simulink model "trainn_traction_system_4motors_CRH3_ver1"  (R2020b)
settings: Solver=VariableStepAuto  StartTime=0.0  StopTime=3  RelTol=1e-3
model workspace (MAT data in the model file):
  C = 0.016
  J = 5
  L = 0.005
  Llr = 0.006
  Lls = 0.001416
  Lm = 0.0254
  R = 0.2
  Rr = 0.16
  Rs = 0.15
  T = 1e-06
  Tloadmax = 100
  Tloadstart = 2
  Tpwm = 0.0001
  Ts = 0.0008
  Vdc_ref = 2700
  Vpeak = 1550
  f = 50
  noiseDense = 0.01
  np = 2
  sample_time = 2e-05
  tE1 = 3.25
  tE1w = 10
  tE2 = 10
  tE2w = 10
  tE3 = 10
  tE3w = 10
  tE4 = 10
  tE4w = 10
  t_precharge = 0.15
  w = 314.159265359
libraries: powerlib x19, simulink x19, pid_lib x1, eeSinusoidalMeasurementV2 x1
(part 1 of 3)
settings Model: SimulationMode=accelerator  OrderedModelArguments=off  Creator=messer  LastModifiedBy=messer

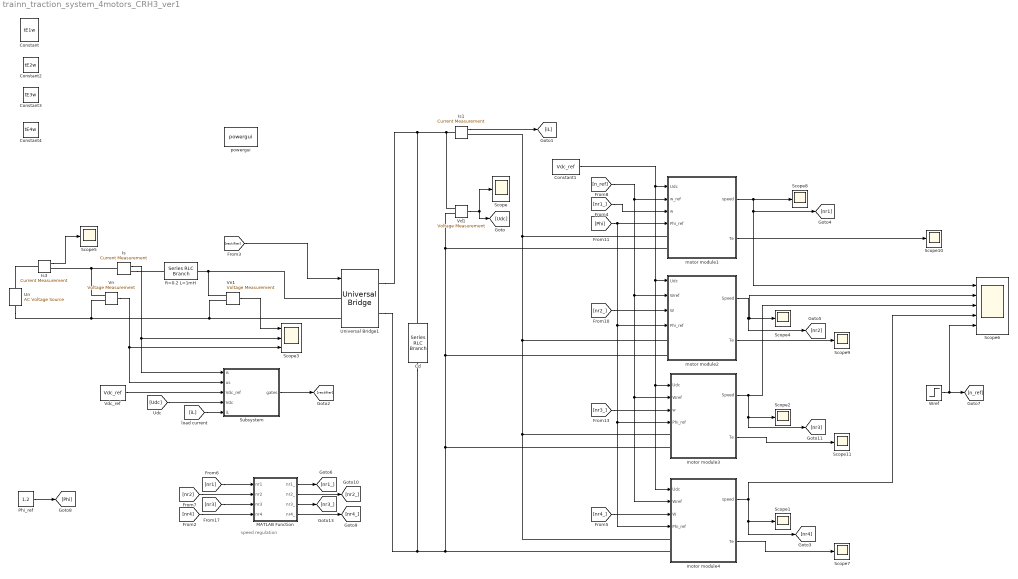
== system trainn_traction_system_4motors_CRH3_ver1 ==
  note: speed regulation
  Cd : powerlib/Elements/Series RLC Branch  LConnTagsString=__new0  RConnTagsString=__new0  BranchType=C  Resistance=1  Inductance=1e-3  SetiL0=off  InitialCurrent=0  Capacitance=C  Setx0=off  InitialVoltage=0  Measurements=None
  Constant : Constant  Value=tE1w
  Constant1 : Constant  Value=Vdc_ref
  Constant2 : Constant  Value=tE2w
  Constant3 : Constant  Value=tE3w
  Constant4 : Constant  Value=tE4w
  Is : powerlib/Measurements/Current Measurement  PhasorSimulation=off  OutputType=Complex  PSBequivalent=0
  Is1 : powerlib/Measurements/Current Measurement  PhasorSimulation=off  OutputType=Complex  PSBequivalent=0
  Is3 : powerlib/Measurements/Current Measurement  PhasorSimulation=off  OutputType=Complex  PSBequivalent=0
  MATLAB Function : MATLAB Function  TreatAsAtomicUnit=on
  Phi_ref : Constant  Value=1.2
  R=0.2 L=1mH : powerlib/Elements/Series RLC Branch  LConnTagsString=__new0  RConnTagsString=__new0  BranchType=RL  Resistance=R  Inductance=L  SetiL0=off  InitialCurrent=0  Capacitance=1e-6  Setx0=off  InitialVoltage=0  Measurements=None
  Scope{,1..2,4..5,7..11} (10 alike) : Scope
  Scope3 : Scope  NumInputPorts=3
  Scope6 : Scope  NumInputPorts=5
  Subsystem : Subsystem
  Un : powerlib/Electrical Sources/AC Voltage Source  Amplitude=Vpeak  Phase=0  Frequency=f  SampleTime=0  Measurements=None  BusType=swing  Pref=10e3  Qref=0  Qmin=-inf  Qmax=+inf
  Universal Bridge1 : powerlib/Power Electronics/Universal Bridge  Arms=2  SnubberResistance=1e5  SnubberCapacitance=inf  Device=IGBT / Diodes  Ron=1e-3  Lon=0  ForwardVoltages="[  0  0  ]"  ForwardVoltage=0  GTOparameters=[ 10e-6 , 20e-6 ]  IGBTparameters=[ 1e-6 , 2e-6 ]  Measurements=None  Measurements_2=None  converterType=Rectifier
  Vd1 : powerlib/Measurements/Voltage Measurement  PhasorSimulation=off  OutputType=Complex  PSBequivalent=0
  Vdc_ref : Constant  Value=Vdc_ref
  Vn : powerlib/Measurements/Voltage Measurement  PhasorSimulation=off  OutputType=Complex  PSBequivalent=0
  Vn1 : powerlib/Measurements/Voltage Measurement  PhasorSimulation=off  OutputType=Complex  PSBequivalent=0
  Wref : Step  Time=10  Before=1500  After=2000  SampleTime=0
  motor module1 : Subsystem
  motor module2 : Subsystem
  motor module3 : Subsystem
  motor module4 : Subsystem
  powergui : powerlib/powergui  Priority=1  SimulationMode=Discrete  SampleTime=T  frequency=60  Iterations=50  frequencyindice=0  Pbase=100e6  ErrMax=1e-4  UnitsV=kV  UnitsW=MW  buscounter=0  FunctionMessages=off  echomessages=off  EnableUseOfTLC=off  CurrentSourceSwitches=off  DisableSnubberDevices=off  DisableRonSwitches=off  DisableVfSwitches=off  DisplayEquations=off  AutomaticDiscreteSolvers=off  SolverType=Tustin/Backward Euler (TBE)  Interpol=off  ExternalGateDelay=off  methode=off  Ts=10  x0status=blocks  SPID=off  SwTol=0  HookPort=off  NonlinearTolerance=1e-4  nMaxIteration=100  ContinueOnMaxIteration=off  RestoreLinks=warning  ResistiveCurrentMeasurement=off  Frange=[0:2:500]  Ylog=off  Xlog=on  ShowGrid=off  save=off  variable=ZData  structure=0  ZoomFFT=off  StartTime=0.0  cycles=1  DisplayStyle=1  fundamental=60  FreqAxis=off  MaxFrequency=1000  frequencyindicesteady=1  RmsSteady=1  display=off
  wires:
  Is1/1 -> [iL]
  Vn/1 -> Subsystem/2(us), Scope3/3
  Is/1 -> Subsystem/1(is), Scope3/2
  Vn1/1 -> Scope3/1
  Vd1/1 -> Scope/1, [Udc]
  Vdc_ref/1 -> Subsystem/3(Vdc_ref)
  [Udc] -> Subsystem/4(Vdc)
  [iL] -> Subsystem/5(iL)
  [rectifier] -> Universal Bridge1/1
  Subsystem/1(gates) -> [rectifier]
  [nr1] -> MATLAB Function/1(nr1)
  Wref/1 -> Scope6/5, [n_ref]
  Phi_ref/1 -> [Phi]
  Is3/1 -> Scope5/1
  MATLAB Function/1(nr1_) -> [nr1_]
  MATLAB Function/2(nr2_) -> [nr2_]
  MATLAB Function/3(nr3_) -> [nr3_]
  Constant1/1 -> motor module4/1(Udc), motor module3/1(Udc), motor module2/1(Udc), motor module1/1(Udc)
  [n_ref] -> motor module4/2(Wref), motor module3/2(Wref), motor module2/2(Wref), motor module1/2(w_ref)
  [nr3_] -> motor module3/3(w)
  [Phi] -> motor module1/4(Phi_ref), motor module2/4(Phi_ref), motor module3/4(Phi_ref), motor module4/4(Phi_ref)
  motor module3/1(Speed) -> [nr3], Scope2/1, Scope6/3
  [nr2_] -> motor module2/3(W)
  motor module2/1(Speed) -> [nr2], Scope6/2, Scope4/1
  [nr1_] -> motor module1/3(w)
  motor module1/1(speed) -> Scope6/1, [nr1], Scope8/1
  motor module4/1(speed) -> Scope1/1, [nr4], Scope6/4
  MATLAB Function/4(nr4_) -> [nr4_]
  [nr4_] -> motor module4/3(W)
  [nr2] -> MATLAB Function/2(nr2)
  [nr3] -> MATLAB Function/3(nr3)
  [nr4] -> MATLAB Function/4(nr4)
  motor module1/2(Te) -> Scope10/1
  motor module2/2(Te) -> Scope9/1
  motor module3/2(Te) -> Scope11/1
  motor module4/2(Te) -> Scope7/1
  connections:
  motor module3/LConn1 -- motor module4/LConn1 -- motor module2/LConn1 -- motor module1/LConn1 -- Is1/RConn1
  Is3/RConn1 -- Is/LConn1 -- Vn/LConn1
  Cd/RConn1 -- Vd1/LConn2 -- motor module1/LConn2 -- motor module2/LConn2 -- motor module3/LConn2 -- motor module4/LConn2 -- Universal Bridge1/RConn2
  Universal Bridge1/LConn1 -- R=0.2 L=1mH/RConn1 -- Vn1/LConn1
  Vn1/LConn2 -- Un/LConn1 -- Vn/LConn2 -- Universal Bridge1/LConn2
  Vd1/LConn1 -- Universal Bridge1/RConn1 -- Cd/LConn1 -- Is1/LConn1
  Is/RConn1 -- R=0.2 L=1mH/LConn1
  Is3/LConn1 -- Un/RConn1

== system trainn_traction_system_4motors_CRH3_ver1/Subsystem ==
  is : Inport
  us : Inport  Port=2
  Vdc_ref : Inport  Port=3
  Vdc : Inport  Port=4
  iL : Inport  Port=5
  Gain : Gain  Gain=2/Vpeak
  Gain1 : Gain  Gain=R
  Gain2 : Gain  Gain=w*L
  Gain4 : Gain
  PID Controller : pid_lib/PID Controller  Controller=PI  Form=Parallel  TimeDomain=Continuous-time  UseExternalTs=off  SampleTime=-1  IntegratorMethod=Forward Euler  FilterMethod=Forward Euler  ControllerParametersSource=internal  P=11  I=0.13  D=0  UseFilter=on  N=100  TunerSelectOption=Transfer Function Based (PID Tuner App)  InitialConditionSource=internal  InitialConditionForIntegrator=0  InitialConditionForFilter=0  DifferentiatorICPrevScaledInput=0  ExternalReset=none  TrackingMode=off  Kt=1  LimitOutput=off  SatLimitsSource=internal  UpperSaturationLimit=inf  LowerSaturationLimit=-inf  LinearizeAsGain=on  AntiWindupMode=none  Kb=1  POutMin=[]  POutMax=[]  IOutMin=[]  IOutMax=[]  DOutMin=[]  DOutMax=[]  NOutMin=[]  NOutMax=[]  SumOutMin=[]  SumOutMax=[]  SaturationOutMin=[]  SaturationOutMax=[]  PParamMin=[]  PParamMax=[]  IParamMin=[]  IParamMax=[]  DParamMin=[]  DParamMax=[]  NParamMin=[]  NParamMax=[]  KbParamMin=[]  KbParamMax=[]  KtParamMin=[]  KtParamMax=[]  KbOutMin=[]  KbOutMax=[]  KtOutMin=[]  KtOutMax=[]  IntegratorOutMin=[]  IntegratorOutMax=[]  FilterOutMin=[]  FilterOutMax=[]  SumI1OutMin=[]  SumI1OutMax=[]  SumI2OutMin=[]  SumI2OutMax=[]  SumI3OutMin=[]  SumI3OutMax=[]  SumI4OutMin=[]  SumI4OutMax=[]  SumDOutMin=[]  SumDOutMax=[]  DifferentiatorOutMin=[]  DifferentiatorOutMax=[]  FilterDiffOutCoefMin=[]  FilterDiffOutCoefMax=[]  ReciprocalOutMin=[]  ReciprocalOutMax=[]  SumDenOutMin=[]  SumDenOutMax=[]  SumNumOutMin=[]  SumNumOutMax=[]  DivideOutMin=[]  DivideOutMax=[]  UdiffTsProdOutMin=[]  UdiffTsProdOutMax=[]  NTsProdOutMin=[]  NTsProdOutMax=[]  UintegralTsProdOutMin=[]  UintegralTsProdOutMax=[]  UngainTsProdOutMin=[]  UngainTsProdOutMax=[]  IntegratorContinuousStateAttributes=''  IntegratorStateMustResolveToSignalObject=off  IntegratorRTWStateStorageClass=Auto  FilterContinuousStateAttributes=''  FilterStateMustResolveToSignalObject=off  FilterRTWStateStorageClass=Auto  ParallelPVariant=InternalParameters  IdealPVariant=Disabled  IVariant=InternalParameters  DVariant=Disabled  IntegratorVariant=Continuous  SatVariant=Disabled  AWVariant=Passthrough  PCopyVariant=Disabled  TRVariant=Disabled  FdbkBlocksVariant=Forward  IdealPFdbkVariant=Disabled  SatFdbkVariant=Disabled  DerivativeFilterVariant=Disabled  NVariant=Disabled  NCopyVariant=Disabled_SignalSpec  FilterICVariant=Disabled  IntegratorICVariant=InternalICs  ExternalResetVariant=Disabled  TRSumVariant=Passthrough  SumFdbkVariant=Disabled  SumVariant=Sum_PI  TsampFilterVariant=InternalTs  TsampNgainVariant=Passthrough  TsampIntegralVariant=Passthrough  ExternalSaturationOutDataTypeStr=Inherit: Same as second input
  Product : Product
  Product1 : Product
  Product2 : Product
  SinCos : Trigonometry  Operator=sincos
  Sinusoidal Measurement (PLL) : eeSinusoidalMeasurementV2/Sinusoidal Measurement (PLL)  Ki_PD=1000  Kp_LF=400  Ki_LF=20000  F0=60  Theta0=0  Mag0=1  Ts=-1
      settings: SourceProductBaseCode=PS
  Sum : Sum  Inputs=|+-
  Sum1 : Sum  Inputs=|++
  Sum2 : Sum  Inputs=+-|--
  Sum9 : Sum  Inputs=-+|
  gen_trigger : Subsystem
  gates : Outport
  wires:
  Sum1/1 -> Product2/2, Product1/2
  SinCos/2 -> Product2/1
  SinCos/1 -> Product1/1
  Gain/1 -> Sum1/2
  Sum/1 -> PID Controller/1
  Vdc/1 -> Product/1, Sum/2
  Product1/1 -> Sum9/2, Gain1/1
  PID Controller/1 -> Sum1/1
  Product/1 -> Gain/1
  Product2/1 -> Gain2/1
  Sinusoidal Measurement (PLL)/2 -> SinCos/1
  Gain2/1 -> Sum2/4
  is/1 -> Sum2/1, Sum9/1
  iL/1 -> Product/2
  Sum2/1 -> gen_trigger/1(uab)
  Gain4/1 -> Sum2/2
  Gain1/1 -> Sum2/3
  Sum9/1 -> Gain4/1
  us/1 -> Sinusoidal Measurement (PLL)/1
  gen_trigger/1(gates) -> gates/1
  Vdc_ref/1 -> Sum/1

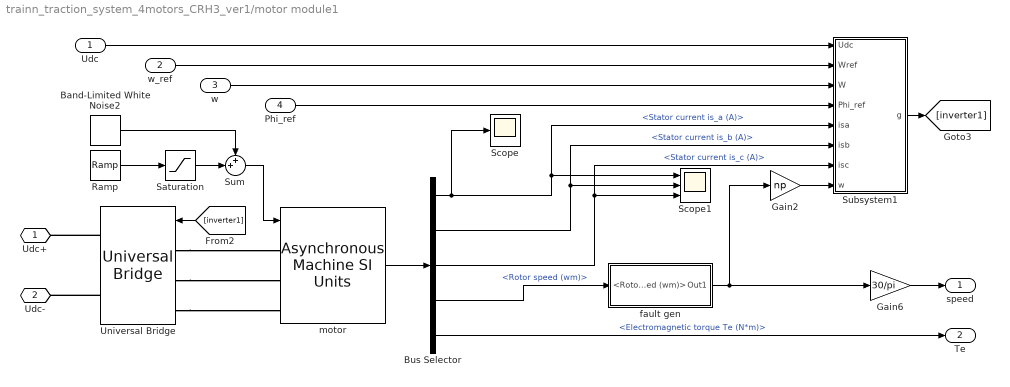
== system trainn_traction_system_4motors_CRH3_ver1/motor module1 ==
  Udc : Inport
  w_ref : Inport  Port=2
  w : Inport  Port=3
  Phi_ref : Inport  Port=4
  Band-Limited White Noise2 : simulink/Sources/Band-Limited White Noise  Cov=[0.0001]  Ts=1e-4  seed=[130341]
  Bus Selector : BusSelector  OutputSignals=Stator measurements.Stator current is_a (A),Stator measurements.Stator current is_b (A),Stator measurements.Stator current is_c (A),Mechanical.Rotor speed (wm),Mechanical.Electromagnetic torque Te (N*m)
  Gain2 : Gain  Gain=np
  Gain6 : Gain  Gain=30/pi
  Ramp : simulink/Sources/Ramp  slope=240  start=Tloadstart  InitialOutput=0
  Saturation : Saturate  UpperLimit=Tloadmax  LowerLimit=0
  Scope : Scope
  Scope1 : Scope  NumInputPorts=3
  Subsystem1 : Subsystem
  Sum : Sum  Inputs=++|
  Universal Bridge : powerlib/Power Electronics/Universal Bridge  Arms=3  SnubberResistance=1e5  SnubberCapacitance=inf  Device=IGBT / Diodes  Ron=1e-3  Lon=0  ForwardVoltages="[  0  0  ]"  ForwardVoltage=0  GTOparameters=[ 10e-6 , 20e-6 ]  IGBTparameters=[ 1e-6 , 2e-6 ]  Measurements=None  Measurements_2=None  converterType=Rectifier
  fault gen : Subsystem
  motor : powerlib/Machines/Asynchronous Machine SI Units  RotorType=Squirrel-cage  PresetModel=No  MechanicalLoad=Torque Tm  ShowDetailedParameters=on  ReferenceFrame=Stationary  Units=SI  MeasurementBus=off  NominalParameters=[562000 2750 135]  Stator=[1.02136*Rs 0.808987*Lls]  Rotor=[0.95069*Rr 0.92145*Llr]  Cage1=[0.4155 0.002066]  Cage2=[0.4168 0.0003495]  Lm=0.88963*Lm  Mechanical=[0.97052*J 0 np]  PolePairs=2  InitialConditions=[1 0 0 0 0 0 0 0]  SimulateSaturation=off  Saturation=[14.03593122, 27.81365428, 53.79336849, 72.68890987, 97.98006896, 148.6815601, 215.7428561, 302.9841135, 428.7778367 ; 230, 322, 414, 460, 506, 552, 598, 644, 690]  LoadFlowParameters=1492000  TsPowergui=0  TsBlock=-1  IterativeModel=Trapezoidal non iterative  IterativeDiscreteModel=Trapezoidal non iterative  Pmec=1.492e+006
  Udc+ : PMIOPort  Side=Left
  Udc- : PMIOPort  Port=2  Side=Left
  speed : Outport
  Te : Outport  Port=2
  wires:
  Gain6/1 -> speed/1
  Subsystem1/1(g) -> [inverter1]
  Bus Selector/1 -> Scope/1, Subsystem1/5(isa), Scope1/1  "<Stator current is_a (A)>"
  Bus Selector/2 -> Subsystem1/6(isb), Scope1/2  "<Stator current is_b (A)>"
  motor/1 -> Bus Selector/1
  Gain2/1 -> Subsystem1/8(w)
  Bus Selector/3 -> Subsystem1/7(isc), Scope1/3  "<Stator current is_c (A)>"
  Bus Selector/5 -> Te/1  "<Electromagnetic torque Te (N*m)>"
  [inverter1] -> Universal Bridge/1
  Udc/1 -> Subsystem1/1(Udc)
  w/1 -> Subsystem1/3(W)
  Phi_ref/1 -> Subsystem1/4(Phi_ref)
  w_ref/1 -> Subsystem1/2(Wref)
  Ramp/1 -> Saturation/1
  Saturation/1 -> Sum/2
  Band-Limited White Noise2/1 -> Sum/1
  Sum/1 -> motor/1
  fault gen/1(Out1) -> Gain6/1, Gain2/1
  Bus Selector/4 -> fault gen/1(<Rotor speed (wm)>)  "<Rotor speed (wm)>"
  connections:
  Universal Bridge/LConn2 -- motor/LConn2
  Universal Bridge/LConn1 -- motor/LConn1
  Universal Bridge/LConn3 -- motor/LConn3
  Universal Bridge/RConn2 -- Udc-/RConn1
  Universal Bridge/RConn1 -- Udc+/RConn1

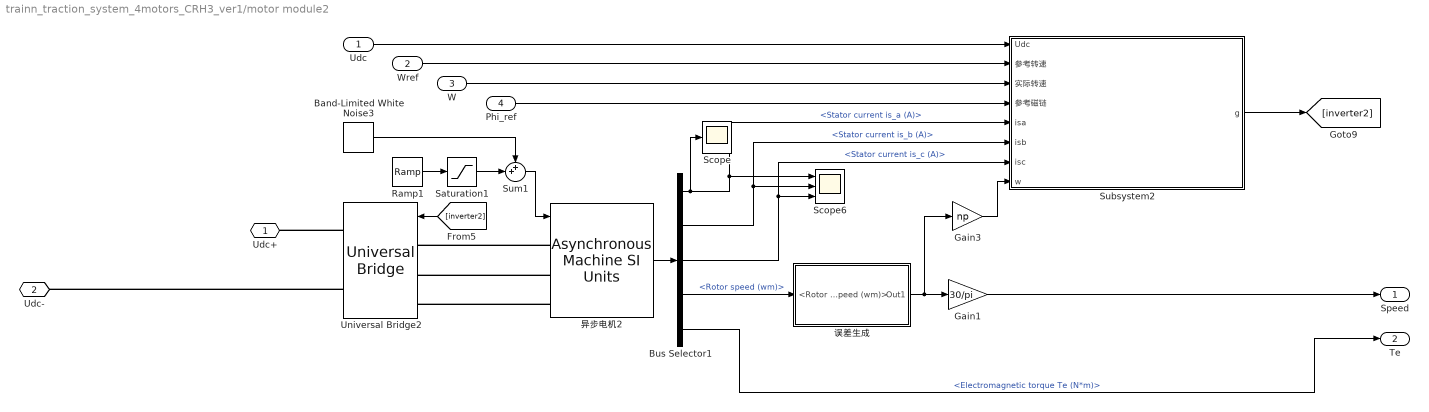
== system trainn_traction_system_4motors_CRH3_ver1/motor module2 ==
  Udc : Inport
  Wref : Inport  Port=2
  W : Inport  Port=3
  Phi_ref : Inport  Port=4
  Band-Limited White Noise3 : simulink/Sources/Band-Limited White Noise  Cov=[0.0001]  Ts=1e-4  seed=[130341]
  Bus Selector1 : BusSelector  OutputSignals=Stator measurements.Stator current is_a (A),Stator measurements.Stator current is_b (A),Stator measurements.Stator current is_c (A),Mechanical.Rotor speed (wm),Mechanical.Electromagnetic torque Te (N*m)
  Gain1 : Gain  Gain=30/pi
  Gain3 : Gain  Gain=np
  Ramp1 : simulink/Sources/Ramp  slope=240  start=Tloadstart  InitialOutput=0
  Saturation1 : Saturate  UpperLimit=Tloadmax  LowerLimit=0
  Scope : Scope
  Scope6 : Scope  NumInputPorts=3
  Subsystem2 : Subsystem
  Sum1 : Sum  Inputs=++|
  Universal Bridge2 : powerlib/Power Electronics/Universal Bridge  Arms=3  SnubberResistance=1e5  SnubberCapacitance=inf  Device=IGBT / Diodes  Ron=1e-3  Lon=0  ForwardVoltages="[  0  0  ]"  ForwardVoltage=0  GTOparameters=[ 10e-6 , 20e-6 ]  IGBTparameters=[ 1e-6 , 2e-6 ]  Measurements=None  Measurements_2=None  converterType=Rectifier
  异步电机2 : powerlib/Machines/Asynchronous Machine SI Units  RotorType=Squirrel-cage  PresetModel=No  MechanicalLoad=Torque Tm  ShowDetailedParameters=on  ReferenceFrame=Stationary  Units=SI  MeasurementBus=off  NominalParameters=[562000 2750 135]  Stator=[1.09135*Rs 0.864431*Lls]  Rotor=[0.9864*Rr 0.92145*Llr]  Cage1=[0.4155 0.002066]  Cage2=[0.4168 0.0003495]  Lm=Lm*1.03442  Mechanical=[1.054266*J 0 np]  PolePairs=2  InitialConditions=[1 0 0 0 0 0 0 0]  SimulateSaturation=off  Saturation=[14.03593122, 27.81365428, 53.79336849, 72.68890987, 97.98006896, 148.6815601, 215.7428561, 302.9841135, 428.7778367 ; 230, 322, 414, 460, 506, 552, 598, 644, 690]  LoadFlowParameters=1492000  TsPowergui=0  TsBlock=-1  IterativeModel=Trapezoidal non iterative  IterativeDiscreteModel=Trapezoidal non iterative  Pmec=1.492e+006
  误差生成 : Subsystem
  Udc+ : PMIOPort  Side=Left
  Udc- : PMIOPort  Port=2  Side=Left
  Speed : Outport
  Te : Outport  Port=2
  wires:
  Bus Selector1/2 -> Subsystem2/6(isb), Scope6/2  "<Stator current is_b (A)>"
  异步电机2/1 -> Bus Selector1/1
  Bus Selector1/4 -> 误差生成/1(<Rotor speed (wm)>)  "<Rotor speed (wm)>"
  W/1 -> Subsystem2/3(实际转速)
  Gain1/1 -> Speed/1
  Bus Selector1/3 -> Subsystem2/7(isc), Scope6/3  "<Stator current is_c (A)>"
  [inverter2] -> Universal Bridge2/1
  Subsystem2/1(g) -> [inverter2]
  Gain3/1 -> Subsystem2/8(w)
  Udc/1 -> Subsystem2/1(Udc)
  Bus Selector1/1 -> Scope/1, Subsystem2/5(isa), Scope6/1  "<Stator current is_a (A)>"
  Bus Selector1/5 -> Te/1  "<Electromagnetic torque Te (N*m)>"
  Phi_ref/1 -> Subsystem2/4(参考磁链)
  Wref/1 -> Subsystem2/2(参考转速)
  误差生成/1(Out1) -> Gain3/1, Gain1/1
  Band-Limited White Noise3/1 -> Sum1/1
  Ramp1/1 -> Saturation1/1
  Saturation1/1 -> Sum1/2
  Sum1/1 -> 异步电机2/1
  connections:
  异步电机2/LConn2 -- Universal Bridge2/LConn2
  异步电机2/LConn1 -- Universal Bridge2/LConn1
  异步电机2/LConn3 -- Universal Bridge2/LConn3
  Universal Bridge2/RConn2 -- Udc-/RConn1
  Universal Bridge2/RConn1 -- Udc+/RConn1

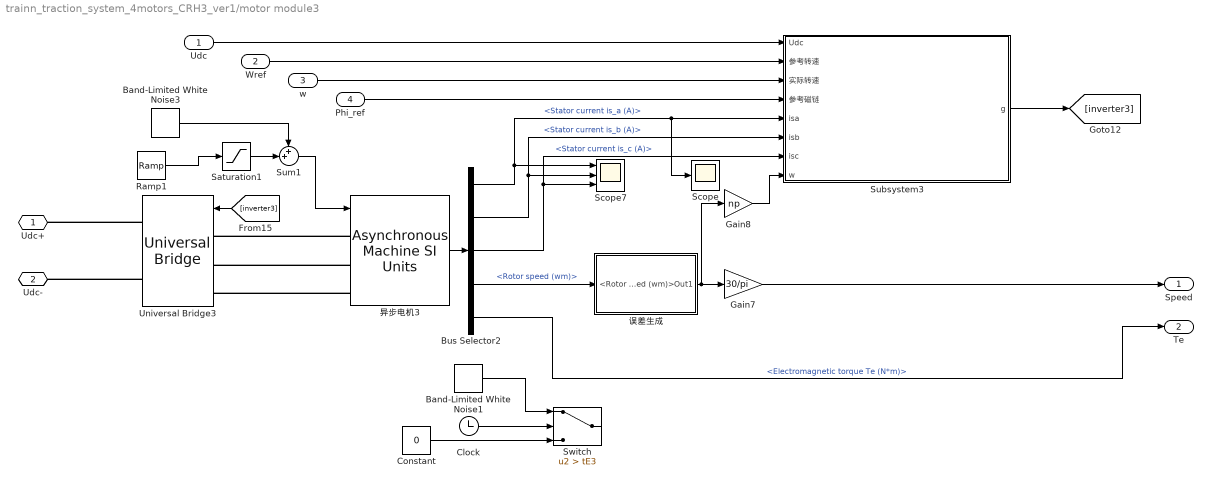
== system trainn_traction_system_4motors_CRH3_ver1/motor module3 ==
  Udc : Inport
  Wref : Inport  Port=2
  w : Inport  Port=3
  Phi_ref : Inport  Port=4
  Band-Limited White Noise1 : simulink/Sources/Band-Limited White Noise  Cov=[0.11]  Ts=noiseDense  seed=[23341]
  Band-Limited White Noise3 : simulink/Sources/Band-Limited White Noise  Cov=[0.0001]  Ts=1e-4  seed=[130341]
  Bus Selector2 : BusSelector  OutputSignals=Stator measurements.Stator current is_a (A),Stator measurements.Stator current is_b (A),Stator measurements.Stator current is_c (A),Mechanical.Rotor speed (wm),Mechanical.Electromagnetic torque Te (N*m)
  Clock : Clock
  Constant : Constant  Value=0
  Gain7 : Gain  Gain=30/pi
  Gain8 : Gain  Gain=np
  Ramp1 : simulink/Sources/Ramp  slope=240  start=Tloadstart  InitialOutput=0
  Saturation1 : Saturate  UpperLimit=Tloadmax  LowerLimit=0
  Scope : Scope
  Scope7 : Scope  NumInputPorts=3
  Subsystem3 : Subsystem
  Sum1 : Sum  Inputs=++|
  Switch : Switch  Criteria=u2 > Threshold  Threshold=tE3
  Universal Bridge3 : powerlib/Power Electronics/Universal Bridge  Arms=3  SnubberResistance=1e5  SnubberCapacitance=inf  Device=IGBT / Diodes  Ron=1e-3  Lon=0  ForwardVoltages="[  0  0  ]"  ForwardVoltage=0  GTOparameters=[ 10e-6 , 20e-6 ]  IGBTparameters=[ 1e-6 , 2e-6 ]  Measurements=None  Measurements_2=None  converterType=Rectifier
  异步电机3 : powerlib/Machines/Asynchronous Machine SI Units  RotorType=Squirrel-cage  PresetModel=No  MechanicalLoad=Torque Tm  ShowDetailedParameters=on  ReferenceFrame=Stationary  Units=SI  MeasurementBus=off  NominalParameters=[562000 2750 135]  Stator=[0.9819810*Rs Lls*0.832368]  Rotor=[0.978836*Rr Llr*1.00113]  Cage1=[0.4155 0.002066]  Cage2=[0.4168 0.0003495]  Lm=Lm*0.938915  Mechanical=[0.98615*J 0 np]  PolePairs=2  InitialConditions=[1 0 0 0 0 0 0 0]  SimulateSaturation=off  Saturation=[14.03593122, 27.81365428, 53.79336849, 72.68890987, 97.98006896, 148.6815601, 215.7428561, 302.9841135, 428.7778367 ; 230, 322, 414, 460, 506, 552, 598, 644, 690]  LoadFlowParameters=1492000  TsPowergui=0  TsBlock=-1  IterativeModel=Trapezoidal non iterative  IterativeDiscreteModel=Trapezoidal non iterative  Pmec=1.492e+006
  误差生成 : Subsystem
  Udc+ : PMIOPort  Side=Left
  Udc- : PMIOPort  Port=2  Side=Left
  Speed : Outport
  Te : Outport  Port=2
  wires:
  Bus Selector2/1 -> Scope/1, Subsystem3/5(isa), Scope7/1  "<Stator current is_a (A)>"
  Bus Selector2/4 -> 误差生成/1(<Rotor speed (wm)>)  "<Rotor speed (wm)>"
  Subsystem3/1(g) -> [inverter3]
  Gain7/1 -> Speed/1
  Bus Selector2/5 -> Te/1  "<Electromagnetic torque Te (N*m)>"
  Bus Selector2/3 -> Scope7/3, Subsystem3/7(isc)  "<Stator current is_c (A)>"
  Wref/1 -> Subsystem3/2(参考转速)
  Gain8/1 -> Subsystem3/8(w)
  [inverter3] -> Universal Bridge3/1
  Bus Selector2/2 -> Subsystem3/6(isb), Scope7/2  "<Stator current is_b (A)>"
  异步电机3/1 -> Bus Selector2/1
  w/1 -> Subsystem3/3(实际转速)
  Phi_ref/1 -> Subsystem3/4(参考磁链)
  Udc/1 -> Subsystem3/1(Udc)
  Band-Limited White Noise1/1 -> Switch/1
  Constant/1 -> Switch/3
  Clock/1 -> Switch/2
  误差生成/1(Out1) -> Gain8/1, Gain7/1
  Band-Limited White Noise3/1 -> Sum1/1
  Ramp1/1 -> Saturation1/1
  Saturation1/1 -> Sum1/2
  Sum1/1 -> 异步电机3/1
  connections:
  异步电机3/LConn1 -- Universal Bridge3/LConn1
  异步电机3/LConn3 -- Universal Bridge3/LConn3
  异步电机3/LConn2 -- Universal Bridge3/LConn2
  Universal Bridge3/RConn1 -- Udc+/RConn1
  Universal Bridge3/RConn2 -- Udc-/RConn1

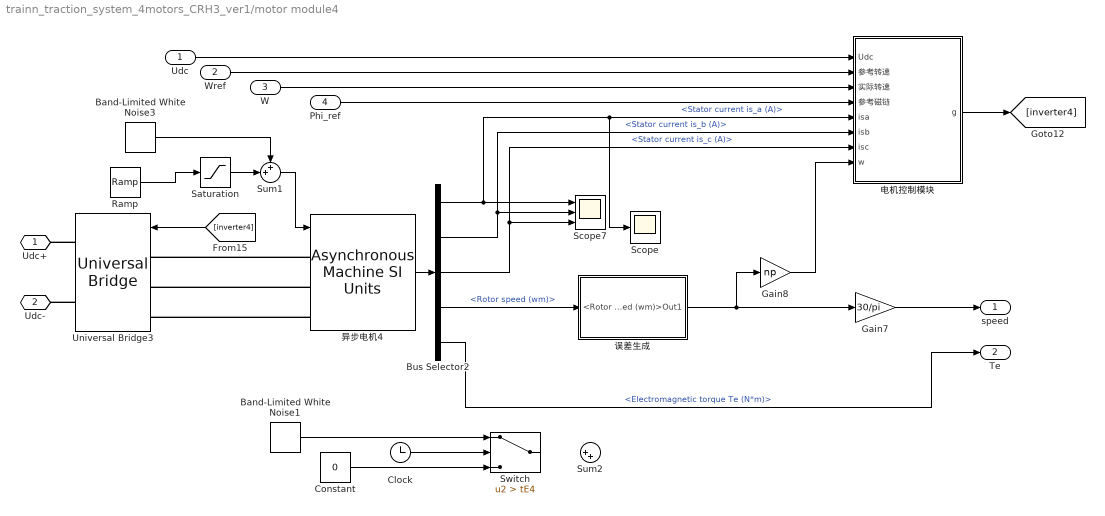
== system trainn_traction_system_4motors_CRH3_ver1/motor module4 ==
  Udc : Inport
  Wref : Inport  Port=2
  W : Inport  Port=3
  Phi_ref : Inport  Port=4
  Band-Limited White Noise1 : simulink/Sources/Band-Limited White Noise  Cov=[0.11]  Ts=noiseDense  seed=[23341]
  Band-Limited White Noise3 : simulink/Sources/Band-Limited White Noise  Cov=[0.0001]  Ts=1e-4  seed=[130341]
  Bus Selector2 : BusSelector  OutputSignals=Stator measurements.Stator current is_a (A),Stator measurements.Stator current is_b (A),Stator measurements.Stator current is_c (A),Mechanical.Rotor speed (wm),Mechanical.Electromagnetic torque Te (N*m)
  Clock : Clock
  Constant : Constant  Value=0
  Gain7 : Gain  Gain=30/pi
  Gain8 : Gain  Gain=np
  Ramp : simulink/Sources/Ramp  slope=240  start=Tloadstart  InitialOutput=0
  Saturation : Saturate  UpperLimit=Tloadmax  LowerLimit=0
  Scope : Scope
  Scope7 : Scope  NumInputPorts=3
  Sum1 : Sum  Inputs=++|
  Sum2 : Sum  Inputs=|++
  Switch : Switch  Criteria=u2 > Threshold  Threshold=tE4
  Universal Bridge3 : powerlib/Power Electronics/Universal Bridge  Arms=3  SnubberResistance=1e5  SnubberCapacitance=inf  Device=IGBT / Diodes  Ron=1e-3  Lon=0  ForwardVoltages="[  0  0  ]"  ForwardVoltage=0  GTOparameters=[ 10e-6 , 20e-6 ]  IGBTparameters=[ 1e-6 , 2e-6 ]  Measurements=None  Measurements_2=None  converterType=Rectifier
  异步电机4 : powerlib/Machines/Asynchronous Machine SI Units  RotorType=Squirrel-cage  PresetModel=No  MechanicalLoad=Torque Tm  ShowDetailedParameters=on  ReferenceFrame=Stationary  Units=SI  MeasurementBus=off  NominalParameters=[562000 2750 135]  Stator=[1.02136*Rs Lls*0.8933278]  Rotor=[1.01302*Rr Llr*1.037898]  Cage1=[0.4155 0.002066]  Cage2=[0.4168 0.0003495]  Lm=Lm*1.00281  Mechanical=[0.97849*J 0 np]  PolePairs=2  InitialConditions=[1 0 0 0 0 0 0 0]  SimulateSaturation=off  Saturation=[14.03593122, 27.81365428, 53.79336849, 72.68890987, 97.98006896, 148.6815601, 215.7428561, 302.9841135, 428.7778367 ; 230, 322, 414, 460, 506, 552, 598, 644, 690]  LoadFlowParameters=1492000  TsPowergui=0  TsBlock=-1  IterativeModel=Trapezoidal non iterative  IterativeDiscreteModel=Trapezoidal non iterative  Pmec=1.492e+006
  电机控制模块 : Subsystem
  误差生成 : Subsystem
  Udc+ : PMIOPort  Side=Left
  Udc- : PMIOPort  Port=2  Side=Left
  speed : Outport
  Te : Outport  Port=2
  wires:
  Udc/1 -> 电机控制模块/1(Udc)
  Phi_ref/1 -> 电机控制模块/4(参考磁链)
  W/1 -> 电机控制模块/3(实际转速)
  异步电机4/1 -> Bus Selector2/1
  Bus Selector2/2 -> 电机控制模块/6(isb), Scope7/2  "<Stator current is_b (A)>"
  [inverter4] -> Universal Bridge3/1
  Gain8/1 -> 电机控制模块/8(w)
  Wref/1 -> 电机控制模块/2(参考转速)
  Bus Selector2/3 -> 电机控制模块/7(isc), Scope7/3  "<Stator current is_c (A)>"
  Bus Selector2/5 -> Te/1  "<Electromagnetic torque Te (N*m)>"
  Gain7/1 -> speed/1
  电机控制模块/1(g) -> [inverter4]
  Bus Selector2/4 -> 误差生成/1(<Rotor speed (wm)>)  "<Rotor speed (wm)>"
  Bus Selector2/1 -> Scope/1, 电机控制模块/5(isa), Scope7/1  "<Stator current is_a (A)>"
  Constant/1 -> Switch/3
  Clock/1 -> Switch/2
  Band-Limited White Noise1/1 -> Switch/1
  误差生成/1(Out1) -> Gain7/1, Gain8/1
  Band-Limited White Noise3/1 -> Sum1/1
  Ramp/1 -> Saturation/1
  Saturation/1 -> Sum1/2
  Sum1/1 -> 异步电机4/1
  connections:
  Universal Bridge3/RConn2 -- Udc-/RConn1
  Universal Bridge3/RConn1 -- Udc+/RConn1
  异步电机4/LConn2 -- Universal Bridge3/LConn2
  异步电机4/LConn3 -- Universal Bridge3/LConn3
  异步电机4/LConn1 -- Universal Bridge3/LConn1

== system trainn_traction_system_4motors_CRH3_ver1/Subsystem/gen_trigger ==
  uab : Inport
  Gain4 : Gain  Gain=1/Vdc_ref
  Gain5 : Gain  Gain=-1
  Mux : Mux
  NOT : Logic  Operator=NOT  IconShape=distinctive  AllPortsSameDT=off  OutDataTypeStr=boolean
  NOT1 : Logic  Operator=NOT  IconShape=distinctive  AllPortsSameDT=off  OutDataTypeStr=boolean
  Relational Operator : RelationalOperator  OutDataTypeStr=boolean  RndMeth=Simplest
  Relational Operator1 : RelationalOperator  OutDataTypeStr=boolean  RndMeth=Simplest
  Repeating Sequence : simulink/Sources/Repeating Sequence  rep_seq_t=[0 Ts/2 Ts]  rep_seq_y=[-1 1 -1]
  gates : Outport
  wires:
  Relational Operator1/1 -> NOT1/1, Mux/3
  Repeating Sequence/1 -> Relational Operator1/2, Relational Operator/2
  Gain4/1 -> Relational Operator/1, Gain5/1
  NOT/1 -> Mux/2
  uab/1 -> Gain4/1
  Relational Operator/1 -> NOT/1, Mux/1
  Mux/1 -> gates/1
  Gain5/1 -> Relational Operator1/1
  NOT1/1 -> Mux/4

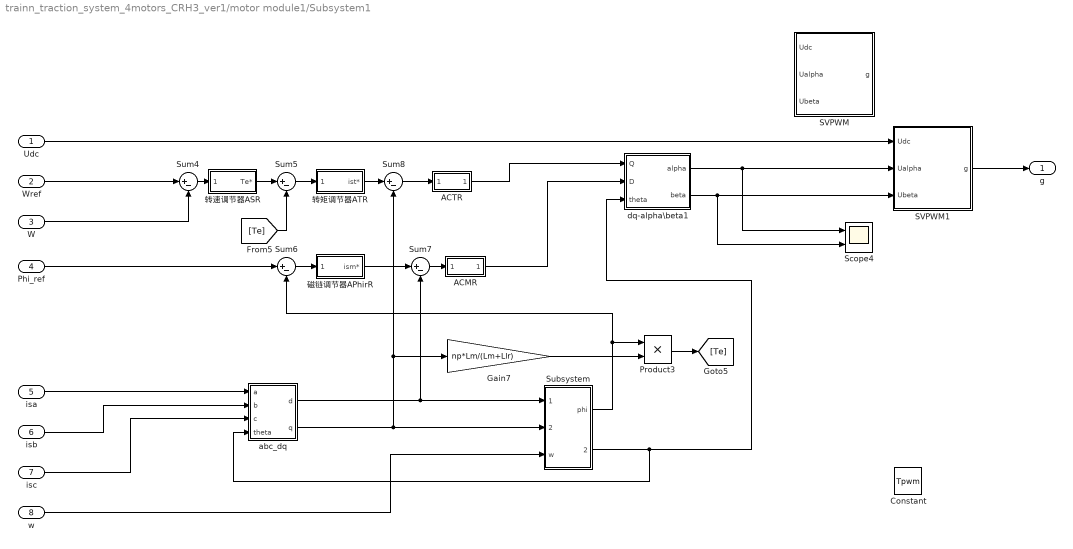
== system trainn_traction_system_4motors_CRH3_ver1/motor module1/Subsystem1 ==
  Udc : Inport
  Wref : Inport  Port=2
  W : Inport  Port=3
  Phi_ref : Inport  Port=4
  isa : Inport  Port=5
  isb : Inport  Port=6
  isc : Inport  Port=7
  w : Inport  Port=8
  ACMR : Subsystem
  ACTR : Subsystem
  Constant : Constant  Value=Tpwm
  Gain7 : Gain  Gain=np*Lm/(Lm+Llr)
  Product3 : Product
  SVPWM : Subsystem
  SVPWM1 : Subsystem
  Scope4 : Scope  NumInputPorts=2
  Subsystem : Subsystem
  Sum{4..8} (5 alike) : Sum  Inputs=|+-
  abc_dq : Subsystem
  dq-alpha\beta1 : Subsystem
  磁链调节器APhirR : Subsystem
  转矩调节器ATR : Subsystem
  转速调节器ASR : Subsystem
  g : Outport
  wires:
  磁链调节器APhirR/1(ism*) -> Sum7/1
  dq-alpha\beta1/1(alpha) -> SVPWM1/2(Ualpha), Scope4/1
  Wref/1 -> Sum4/1
  ACMR/1(" ") -> dq-alpha\beta1/2(D)
  isa/1 -> abc_dq/1(a)
  Sum8/1 -> ACTR/1("  ")
  Subsystem/1(phi) -> Sum6/2, Product3/1
  Subsystem/2(theta) -> abc_dq/4(theta), dq-alpha\beta1/3(theta)
  Gain7/1 -> Product3/2
  W/1 -> Sum4/2
  Product3/1 -> [Te]
  Sum7/1 -> ACMR/1("  ")
  Sum6/1 -> 磁链调节器APhirR/1(" ")
  转矩调节器ATR/1(ist*) -> Sum8/1
  [Te] -> Sum5/2
  转速调节器ASR/1(Te*) -> Sum5/1
  ACTR/1(" ") -> dq-alpha\beta1/1(Q)
  isc/1 -> abc_dq/3(c)
  abc_dq/2(q) -> Subsystem/2(iq(it)), Sum8/2, Gain7/1
  Sum4/1 -> 转速调节器ASR/1("  ")
  abc_dq/1(d) -> Subsystem/1(id(im)), Sum7/2
  dq-alpha\beta1/2(beta) -> SVPWM1/3(Ubeta), Scope4/2
  Sum5/1 -> 转矩调节器ATR/1(" ")
  w/1 -> Subsystem/3(w)
  Phi_ref/1 -> Sum6/1
  isb/1 -> abc_dq/2(b)
  Udc/1 -> SVPWM1/1(Udc)
  SVPWM1/1(g) -> g/1

== system trainn_traction_system_4motors_CRH3_ver1/motor module1/fault gen ==
  <Rotor speed (wm)> : Inport
  Band-Limited White Noise1 : simulink/Sources/Band-Limited White Noise  Cov=[0.11]  Ts=noiseDense  seed=[23341]
  Clock : Clock
  Gain : Gain  Gain=0.9
  Sum2 : Sum  Inputs=++|
  Switch : Switch  Criteria=u2 > Threshold  Threshold=tE1w
  Out1 : Outport
  wires:
  Clock/1 -> Switch/2
  Switch/1 -> Out1/1
  Sum2/1 -> Switch/1
  <Rotor speed (wm)>/1 -> Switch/3, Gain/1
  Band-Limited White Noise1/1 -> Sum2/1
  Gain/1 -> Sum2/2

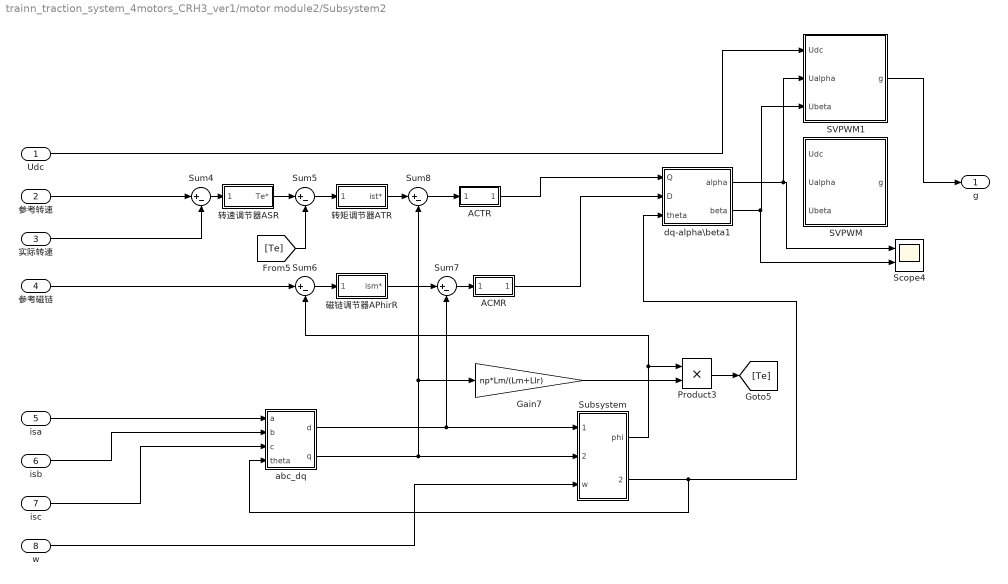
== system trainn_traction_system_4motors_CRH3_ver1/motor module2/Subsystem2 ==
  Udc : Inport
  参考转速 : Inport  Port=2
  实际转速 : Inport  Port=3
  参考磁链 : Inport  Port=4
  isa : Inport  Port=5
  isb : Inport  Port=6
  isc : Inport  Port=7
  w : Inport  Port=8
  ACMR : Subsystem
  ACTR : Subsystem
  Gain7 : Gain  Gain=np*Lm/(Lm+Llr)
  Product3 : Product
  SVPWM : Subsystem
  SVPWM1 : Subsystem
  Scope4 : Scope  NumInputPorts=2
  Subsystem : Subsystem
  Sum{4..8} (5 alike) : Sum  Inputs=|+-
  abc_dq : Subsystem
  dq-alpha\beta1 : Subsystem
  磁链调节器APhirR : Subsystem
  转矩调节器ATR : Subsystem
  转速调节器ASR : Subsystem
  g : Outport
  wires:
  磁链调节器APhirR/1(ism*) -> Sum7/1
  dq-alpha\beta1/1(alpha) -> SVPWM1/2(Ualpha), Scope4/1
  参考转速/1 -> Sum4/1
  ACMR/1(" ") -> dq-alpha\beta1/2(D)
  isa/1 -> abc_dq/1(a)
  Sum8/1 -> ACTR/1("  ")
  Subsystem/1(phi) -> Sum6/2, Product3/1
  Subsystem/2(theta) -> abc_dq/4(theta), dq-alpha\beta1/3(theta)
  Gain7/1 -> Product3/2
  实际转速/1 -> Sum4/2
  Product3/1 -> [Te]
  Sum7/1 -> ACMR/1("  ")
  Sum6/1 -> 磁链调节器APhirR/1(" ")
  转矩调节器ATR/1(ist*) -> Sum8/1
  [Te] -> Sum5/2
  转速调节器ASR/1(Te*) -> Sum5/1
  ACTR/1(" ") -> dq-alpha\beta1/1(Q)
  isc/1 -> abc_dq/3(c)
  abc_dq/2(q) -> Subsystem/2(iq(it)), Sum8/2, Gain7/1
  Sum4/1 -> 转速调节器ASR/1("  ")
  abc_dq/1(d) -> Subsystem/1(id(im)), Sum7/2
  dq-alpha\beta1/2(beta) -> Scope4/2, SVPWM1/3(Ubeta)
  Sum5/1 -> 转矩调节器ATR/1(" ")
  w/1 -> Subsystem/3(w)
  参考磁链/1 -> Sum6/1
  isb/1 -> abc_dq/2(b)
  Udc/1 -> SVPWM1/1(Udc)
  SVPWM1/1(g) -> g/1

== system trainn_traction_system_4motors_CRH3_ver1/motor module2/误差生成 ==
  <Rotor speed (wm)> : Inport
  Band-Limited White Noise1 : simulink/Sources/Band-Limited White Noise  Cov=[0.11]  Ts=noiseDense  seed=[23341]
  Clock : Clock
  Gain : Gain  Gain=0.9
  Sum2 : Sum  Inputs=++|
  Switch : Switch  Criteria=u2 > Threshold  Threshold=tE2w
  Out1 : Outport
  wires:
  Clock/1 -> Switch/2
  Switch/1 -> Out1/1
  Sum2/1 -> Switch/1
  <Rotor speed (wm)>/1 -> Switch/3, Gain/1
  Band-Limited White Noise1/1 -> Sum2/1
  Gain/1 -> Sum2/2

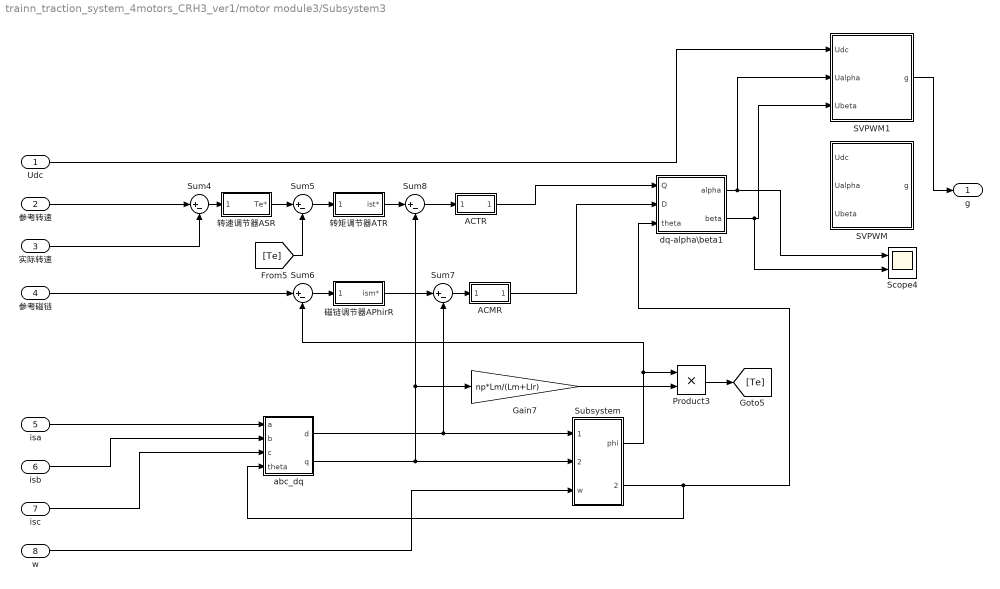
== system trainn_traction_system_4motors_CRH3_ver1/motor module3/Subsystem3 ==
  Udc : Inport
  参考转速 : Inport  Port=2
  实际转速 : Inport  Port=3
  参考磁链 : Inport  Port=4
  isa : Inport  Port=5
  isb : Inport  Port=6
  isc : Inport  Port=7
  w : Inport  Port=8
  ACMR : Subsystem
  ACTR : Subsystem
  Gain7 : Gain  Gain=np*Lm/(Lm+Llr)
  Product3 : Product
  SVPWM : Subsystem
  SVPWM1 : Subsystem
  Scope4 : Scope  NumInputPorts=2
  Subsystem : Subsystem
  Sum{4..8} (5 alike) : Sum  Inputs=|+-
  abc_dq : Subsystem
  dq-alpha\beta1 : Subsystem
  磁链调节器APhirR : Subsystem
  转矩调节器ATR : Subsystem
  转速调节器ASR : Subsystem
  g : Outport
  wires:
  磁链调节器APhirR/1(ism*) -> Sum7/1
  dq-alpha\beta1/1(alpha) -> SVPWM1/2(Ualpha), Scope4/1
  参考转速/1 -> Sum4/1
  ACMR/1(" ") -> dq-alpha\beta1/2(D)
  isa/1 -> abc_dq/1(a)
  Sum8/1 -> ACTR/1("  ")
  Subsystem/1(phi) -> Sum6/2, Product3/1
  Subsystem/2(theta) -> abc_dq/4(theta), dq-alpha\beta1/3(theta)
  Gain7/1 -> Product3/2
  实际转速/1 -> Sum4/2
  Product3/1 -> [Te]
  Sum7/1 -> ACMR/1("  ")
  Sum6/1 -> 磁链调节器APhirR/1(" ")
  转矩调节器ATR/1(ist*) -> Sum8/1
  [Te] -> Sum5/2
  转速调节器ASR/1(Te*) -> Sum5/1
  ACTR/1(" ") -> dq-alpha\beta1/1(Q)
  isc/1 -> abc_dq/3(c)
  abc_dq/2(q) -> Subsystem/2(iq(it)), Sum8/2, Gain7/1
  Sum4/1 -> 转速调节器ASR/1("  ")
  abc_dq/1(d) -> Subsystem/1(id(im)), Sum7/2
  dq-alpha\beta1/2(beta) -> Scope4/2, SVPWM1/3(Ubeta)
  Sum5/1 -> 转矩调节器ATR/1(" ")
  w/1 -> Subsystem/3(w)
  参考磁链/1 -> Sum6/1
  isb/1 -> abc_dq/2(b)
  Udc/1 -> SVPWM1/1(Udc)
  SVPWM1/1(g) -> g/1

== system trainn_traction_system_4motors_CRH3_ver1/motor module3/误差生成 ==
  <Rotor speed (wm)> : Inport
  Band-Limited White Noise1 : simulink/Sources/Band-Limited White Noise  Cov=[0.11]  Ts=noiseDense  seed=[781341]
  Clock : Clock
  Gain : Gain  Gain=0.9
  Sum2 : Sum  Inputs=++|
  Switch : Switch  Criteria=u2 > Threshold  Threshold=tE3w
  Out1 : Outport
  wires:
  Clock/1 -> Switch/2
  Switch/1 -> Out1/1
  Sum2/1 -> Switch/1
  <Rotor speed (wm)>/1 -> Switch/3, Gain/1
  Band-Limited White Noise1/1 -> Sum2/1
  Gain/1 -> Sum2/2

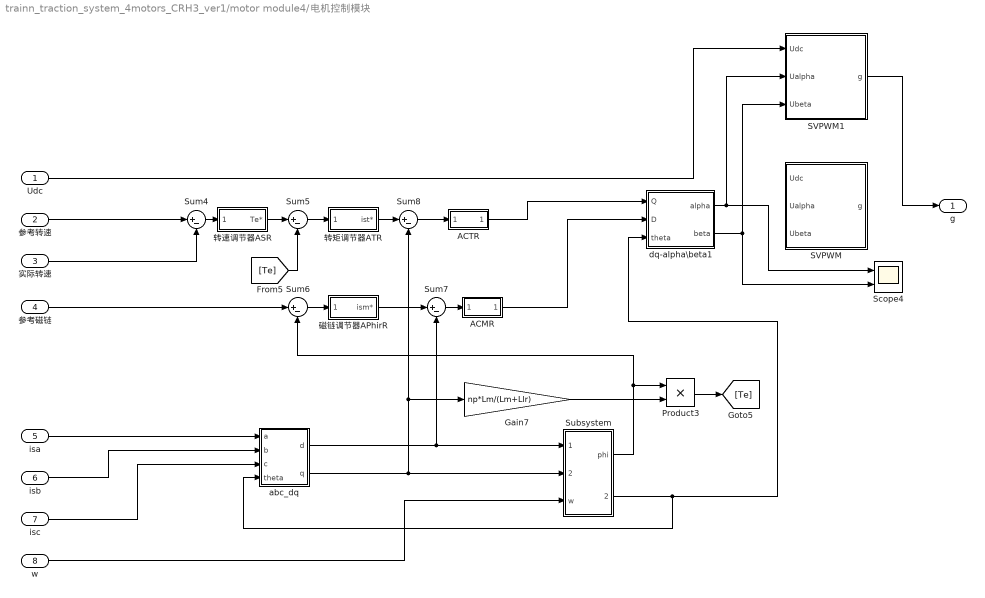
== system trainn_traction_system_4motors_CRH3_ver1/motor module4/电机控制模块 ==
  Udc : Inport
  参考转速 : Inport  Port=2
  实际转速 : Inport  Port=3
  参考磁链 : Inport  Port=4
  isa : Inport  Port=5
  isb : Inport  Port=6
  isc : Inport  Port=7
  w : Inport  Port=8
  ACMR : Subsystem
  ACTR : Subsystem
  Gain7 : Gain  Gain=np*Lm/(Lm+Llr)
  Product3 : Product
  SVPWM : Subsystem
  SVPWM1 : Subsystem
  Scope4 : Scope  NumInputPorts=2
  Subsystem : Subsystem
  Sum{4..8} (5 alike) : Sum  Inputs=|+-
  abc_dq : Subsystem
  dq-alpha\beta1 : Subsystem
  磁链调节器APhirR : Subsystem
  转矩调节器ATR : Subsystem
  转速调节器ASR : Subsystem
  g : Outport
  wires:
  Udc/1 -> SVPWM1/1(Udc)
  isb/1 -> abc_dq/2(b)
  参考磁链/1 -> Sum6/1
  w/1 -> Subsystem/3(w)
  Sum5/1 -> 转矩调节器ATR/1(" ")
  dq-alpha\beta1/2(beta) -> Scope4/2, SVPWM1/3(Ubeta)
  abc_dq/1(d) -> Sum7/2, Subsystem/1(id(im))
  Sum4/1 -> 转速调节器ASR/1("  ")
  abc_dq/2(q) -> Gain7/1, Sum8/2, Subsystem/2(iq(it))
  isc/1 -> abc_dq/3(c)
  ACTR/1(" ") -> dq-alpha\beta1/1(Q)
  转速调节器ASR/1(Te*) -> Sum5/1
  [Te] -> Sum5/2
  转矩调节器ATR/1(ist*) -> Sum8/1
  Sum6/1 -> 磁链调节器APhirR/1(" ")
  Sum7/1 -> ACMR/1("  ")
  Product3/1 -> [Te]
  实际转速/1 -> Sum4/2
  Gain7/1 -> Product3/2
  Subsystem/2(theta) -> dq-alpha\beta1/3(theta), abc_dq/4(theta)
  Subsystem/1(phi) -> Product3/1, Sum6/2
  Sum8/1 -> ACTR/1("  ")
  isa/1 -> abc_dq/1(a)
  ACMR/1(" ") -> dq-alpha\beta1/2(D)
  参考转速/1 -> Sum4/1
  dq-alpha\beta1/1(alpha) -> SVPWM1/2(Ualpha), Scope4/1
  磁链调节器APhirR/1(ism*) -> Sum7/1
  SVPWM1/1(g) -> g/1

== system trainn_traction_system_4motors_CRH3_ver1/motor module4/误差生成 ==
  <Rotor speed (wm)> : Inport
  Band-Limited White Noise1 : simulink/Sources/Band-Limited White Noise  Cov=[0.11]  Ts=noiseDense  seed=[923641]
  Clock : Clock
  Gain : Gain  Gain=0.9
  Sum2 : Sum  Inputs=++|
  Switch : Switch  Criteria=u2 > Threshold  Threshold=tE4w
  Out1 : Outport
  wires:
  Clock/1 -> Switch/2
  Switch/1 -> Out1/1
  Sum2/1 -> Switch/1
  <Rotor speed (wm)>/1 -> Switch/3, Gain/1
  Band-Limited White Noise1/1 -> Sum2/1
  Gain/1 -> Sum2/2

== system trainn_traction_system_4motors_CRH3_ver1/motor module1/Subsystem1/ACMR ==
  "  " : Inport
  Integrator : Integrator
  I积分放大倍数 : Gain  Gain=50
  PI输出限幅 : Saturate  UpperLimit=Vdc_ref/sqrt(6)  LowerLimit=-Vdc_ref/sqrt(6)
  P比例放大倍数 : Gain
  Scope : Scope  NumInputPorts=2
  Sum1 : Sum  Inputs=|++
  带限幅的连续积分1 : Integrator  LimitOutput=on  UpperSaturationLimit=390  LowerSaturationLimit=-390
  " " : Outport  VectorParamsAs1DForOutWhenUnconnected=off
  wires:
  Sum1/1 -> PI输出限幅/1
  PI输出限幅/1 -> " "/1, Scope/1
  P比例放大倍数/1 -> Sum1/1
  I积分放大倍数/1 -> Integrator/1
  "  "/1 -> I积分放大倍数/1, P比例放大倍数/1
  Integrator/1 -> Scope/2, Sum1/2

== system trainn_traction_system_4motors_CRH3_ver1/motor module1/Subsystem1/ACTR ==
  "  " : Inport
  Integrator : Integrator
  I积分放大倍数 : Gain  Gain=3.5
  PI输出限幅 : Saturate  UpperLimit=Vdc_ref/sqrt(6)  LowerLimit=-1*Vdc_ref/sqrt(6)
  PI输出限幅1 : Saturate  UpperLimit=Vdc_ref  LowerLimit=-1*Vdc_ref
  P比例放大倍数 : Gain  Gain=1.5
  Scope : Scope  NumInputPorts=2
  Sum1 : Sum  Inputs=|++
  带限幅的连续积分1 : Integrator  LimitOutput=on  UpperSaturationLimit=400  LowerSaturationLimit=-400
  " " : Outport  VectorParamsAs1DForOutWhenUnconnected=off
  wires:
  Sum1/1 -> PI输出限幅/1
  PI输出限幅/1 -> " "/1, Scope/1
  P比例放大倍数/1 -> Sum1/1
  I积分放大倍数/1 -> Integrator/1
  "  "/1 -> I积分放大倍数/1, P比例放大倍数/1
  Integrator/1 -> Scope/2, Sum1/2

== system trainn_traction_system_4motors_CRH3_ver1/motor module1/Subsystem1/SVPWM ==
  Udc : Inport
  Ualpha : Inport  Port=2
  Ubeta : Inport  Port=3
  " Gen Gate" : MATLAB Function  TreatAsAtomicUnit=on
  Clock : Clock
  Constant2 : Constant  Value=Ts
  Constant3 : Constant  Value=Ts
  Data Type Conversion : DataTypeConversion  OutDataTypeStr=boolean
  Delay{,1..4} (5 alike) : Delay  DelayLength=1  InitialCondition=0
  MATLAB Function1 : MATLAB Function  TreatAsAtomicUnit=on
  MATLAB Function3 : MATLAB Function  TreatAsAtomicUnit=on
  Pulse Generator : DiscretePulseGenerator  PulseType=Time based  Period=Ts
  Scope1 : Scope  NumInputPorts=3
  Scope3 : Scope
  find section1 : Subsystem
  g : Outport
  wires:
  Ualpha/1 -> find section1/1(Ualpha), MATLAB Function3/2(Ualpha)
  Pulse Generator/1 -> Data Type Conversion/1
  MATLAB Function1/2(newT0) -> " Gen Gate"/4(T0), Delay/1
  Delay1/1 -> MATLAB Function1/1(old_t0)
  MATLAB Function3/3(T2) -> Scope1/3, MATLAB Function1/6(T2)
  Ubeta/1 -> find section1/2(Ubeta), MATLAB Function3/3(Ubeta)
  find section1/1(section) -> MATLAB Function1/7(sec), MATLAB Function3/5(sec)
  Constant2/1 -> MATLAB Function3/4(Ts)
  MATLAB Function3/2(T1) -> Scope1/2, MATLAB Function1/5(T1)
  MATLAB Function1/1(new_t0) -> Scope3/1, Delay1/1, " Gen Gate"/2(t0)
  Clock/1 -> " Gen Gate"/1(t), MATLAB Function1/2(t)
  MATLAB Function3/1(T0) -> MATLAB Function1/4(T0), Scope1/1
  Constant3/1 -> " Gen Gate"/3(Ts)
  Udc/1 -> MATLAB Function3/1(Udc)
  " Gen Gate"/1(g) -> g/1
  Data Type Conversion/1 -> MATLAB Function1/3(trigger)
  MATLAB Function1/5(newSec) -> Delay2/1, " Gen Gate"/7(sec)
  Delay2/1 -> MATLAB Function1/11(oldSec)
  MATLAB Function1/4(newT2) -> Delay3/1, " Gen Gate"/6(T2)
  Delay3/1 -> MATLAB Function1/10(oldT2)
  MATLAB Function1/3(newT1) -> Delay4/1, " Gen Gate"/5(T1)
  Delay4/1 -> MATLAB Function1/9(oldT1)
  Delay/1 -> MATLAB Function1/8(oldT0)

== system trainn_traction_system_4motors_CRH3_ver1/motor module1/Subsystem1/SVPWM1 ==
  Udc : Inport
  Ualpha : Inport  Port=2
  Ubeta : Inport  Port=3
  Constant2 : Constant  Value=Tpwm
  Constant4 : Constant  Value=Tpwm
  MATLAB Function10 : MATLAB Function  TreatAsAtomicUnit=on
  MATLAB Function3 : MATLAB Function  TreatAsAtomicUnit=on
  Mux : Mux  Inputs=6
  Repeating Sequence1 : simulink/Sources/Repeating Sequence  rep_seq_t=[0 Tpwm]  rep_seq_y=[0 Tpwm]
  Scope1 : Scope  NumInputPorts=3
  find section1 : Subsystem
  g : Outport
  wires:
  Ualpha/1 -> find section1/1(Ualpha), MATLAB Function3/2(Ualpha)
  Ubeta/1 -> find section1/2(Ubeta), MATLAB Function3/3(Ubeta)
  Constant2/1 -> MATLAB Function3/4(Ts)
  MATLAB Function3/1(T0) -> Scope1/1
  Udc/1 -> MATLAB Function3/1(Udc)
  MATLAB Function3/2(T1) -> Scope1/2, MATLAB Function10/1(Ta)
  find section1/1(section) -> MATLAB Function10/4(section), MATLAB Function3/5(sec)
  Constant4/1 -> MATLAB Function10/3(Tpwm)
  Repeating Sequence1/1 -> MATLAB Function10/5(t)
  MATLAB Function3/3(T2) -> Scope1/3, MATLAB Function10/2(Tb)
  MATLAB Function10/6(gCN) -> Mux/6
  MATLAB Function10/5(gC) -> Mux/5
  MATLAB Function10/4(gBN) -> Mux/4
  MATLAB Function10/3(gB) -> Mux/3
  MATLAB Function10/2(gAN) -> Mux/2
  MATLAB Function10/1(gA) -> Mux/1
  Mux/1 -> g/1

== system trainn_traction_system_4motors_CRH3_ver1/motor module1/Subsystem1/Subsystem ==
  note: Tr = Lr / Rr
  note: phy_r
  note: ws
  note: w1
  id(im) : Inport
  iq(it) : Inport  Port=2
  w : Inport  Port=3
  Divide{,2..4} (4 alike) : Product  Inputs=/*
  Divide1 : Product  Inputs=*/
  Gain1 : Gain  Gain=Lm
  Gain2 : Gain  Gain=Lm
  Integrator1 : Integrator  InitialCondition=1e-5
  Integrator2 : Integrator
  Lr : Constant  Value=Llr + 1.5*Lm
  Rr : Constant  Value=Rr
  Scope3 : Scope  NumInputPorts=2
  Sum : Sum  Inputs=-+|
  Sum1 : Sum  Inputs=|++
  phi : Outport
  theta : Outport  Port=2
  wires:
  Divide/1 -> Sum1/1
  Divide3/1 -> Divide/2
  Sum/1 -> Integrator1/1
  iq(it)/1 -> Gain2/1, Scope3/2
  Sum1/1 -> Integrator2/1
  id(im)/1 -> Gain1/1, Scope3/1
  w/1 -> Sum1/2
  Integrator2/1 -> theta/1
  Lr/1 -> Divide1/1
  Rr/1 -> Divide1/2
  Divide2/1 -> Sum/2
  Gain1/1 -> Divide2/2
  Integrator1/1 -> Divide4/2, Divide/1, phi/1
  Divide4/1 -> Sum/1
  Divide1/1 -> Divide3/1, Divide2/1, Divide4/1
  Gain2/1 -> Divide3/2

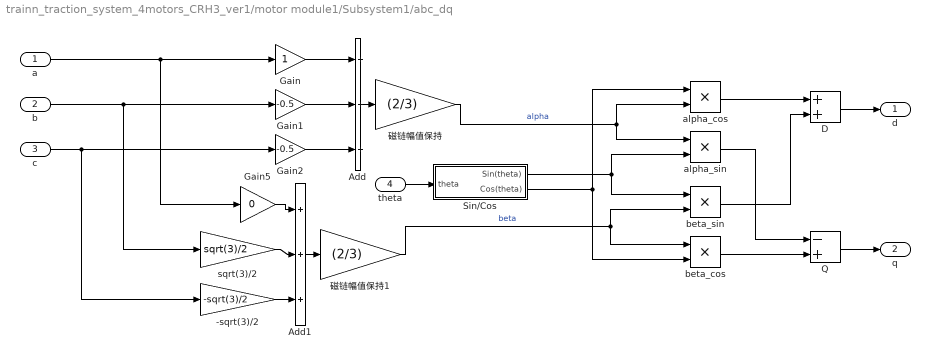
== system trainn_traction_system_4motors_CRH3_ver1/motor module1/Subsystem1/abc_dq ==
  a : Inport
  b : Inport  Port=2
  c : Inport  Port=3
  theta : Inport  Port=4
  -sqrt(3)/2 : Gain  Gain=-sqrt(3)/2
  Add : Sum  Inputs=3
  Add1 : Sum  Inputs=3
  D : Sum
  Gain : Gain
  Gain1 : Gain  Gain=-0.5
  Gain2 : Gain  Gain=-0.5
  Gain5 : Gain  Gain=0
  Q : Sum  Inputs=-+
  Sin/Cos : Subsystem
  alpha_cos : Product
  alpha_sin : Product
  beta_cos : Product
  beta_sin : Product
  sqrt(3)/2 : Gain  Gain=sqrt(3)/2
  磁链幅值保持 : Gain  Gain=(2/3)
  磁链幅值保持1 : Gain  Gain=(2/3)
  d : Outport  VectorParamsAs1DForOutWhenUnconnected=off
  q : Outport  Port=2  VectorParamsAs1DForOutWhenUnconnected=off
  wires:
  磁链幅值保持1/1 -> beta_cos/1, beta_sin/2  "beta"
  D/1 -> d/1
  Sin/Cos/2(Cos(theta)) -> beta_cos/2, alpha_cos/1
  alpha_sin/1 -> Q/1
  Q/1 -> q/1
  beta_sin/1 -> D/2
  beta_cos/1 -> Q/2
  Sin/Cos/1(Sin(theta)) -> beta_sin/1, alpha_sin/2
  磁链幅值保持/1 -> alpha_cos/2, alpha_sin/1  "alpha"
  Add1/1 -> 磁链幅值保持1/1
  c/1 -> Gain2/1, -sqrt(3)/2/1
  a/1 -> Gain5/1, Gain/1
  Gain2/1 -> Add/3
  sqrt(3)/2/1 -> Add1/2
  theta/1 -> Sin/Cos/1(theta)
  b/1 -> sqrt(3)/2/1, Gain1/1
  -sqrt(3)/2/1 -> Add1/3
  Gain1/1 -> Add/2
  Gain5/1 -> Add1/1
  alpha_cos/1 -> D/1
  Add/1 -> 磁链幅值保持/1
  Gain/1 -> Add/1

== system trainn_traction_system_4motors_CRH3_ver1/motor module1/Subsystem1/dq-alpha\beta1 ==
  Q : Inport
  D : Inport  Port=2
  theta : Inport  Port=3
  Product{,1..3} (4 alike) : Product
  Sum1 : Sum  Inputs=++|
  Sum3 : Sum  Inputs=|+-
  Trigonometric Function : Trigonometry
  Trigonometric Function1 : Trigonometry  Operator=cos
  alpha : Outport
  beta : Outport  Port=2
  wires:
  Sum1/1 -> beta/1
  Product3/1 -> Sum1/2
  Product2/1 -> Sum1/1
  Sum3/1 -> alpha/1
  Product1/1 -> Sum3/2
  Product/1 -> Sum3/1
  Trigonometric Function/1 -> Product1/1, Product2/1
  Trigonometric Function1/1 -> Product/2, Product3/1
  Q/1 -> Product1/2, Product3/2
  theta/1 -> Trigonometric Function/1, Trigonometric Function1/1
  D/1 -> Product2/2, Product/1

== system trainn_traction_system_4motors_CRH3_ver1/motor module1/Subsystem1/磁链调节器APhirR ==
  " " : Inport
  Integrator : Integrator
  I积分放大倍数 : Gain  Gain=3.6
  PI输出限幅1 : Saturate  UpperLimit=13  LowerLimit=-13
  P比例放大倍数 : Gain  Gain=1.8
  Scope : Scope  NumInputPorts=2
  Sum1 : Sum  Inputs=|++
  带限幅的连续积分1 : Integrator  LimitOutput=on  UpperSaturationLimit=15  LowerSaturationLimit=-15
  ism* : Outport  VectorParamsAs1DForOutWhenUnconnected=off
  wires:
  P比例放大倍数/1 -> Sum1/1
  " "/1 -> I积分放大倍数/1, P比例放大倍数/1
  Sum1/1 -> ism*/1, Scope/1
  I积分放大倍数/1 -> Integrator/1
  Integrator/1 -> Scope/2, Sum1/2

== system trainn_traction_system_4motors_CRH3_ver1/motor module1/Subsystem1/转矩调节器ATR ==
  " " : Inport
  Integrator : Integrator
  I积分放大倍数 : Gain  Gain=1.1
  PI输出限幅1 : Saturate  UpperLimit=600  LowerLimit=-600
  P比例放大倍数 : Gain  Gain=1.6
  Scope : Scope  NumInputPorts=2
  Sum3 : Sum  Inputs=|++
  带限幅的连续积分1 : Integrator  LimitOutput=on  UpperSaturationLimit=65  LowerSaturationLimit=-65
  ist* : Outport  VectorParamsAs1DForOutWhenUnconnected=off
  wires:
  " "/1 -> I积分放大倍数/1, P比例放大倍数/1
  I积分放大倍数/1 -> Integrator/1
  Sum3/1 -> PI输出限幅1/1
  P比例放大倍数/1 -> Sum3/1
  Integrator/1 -> Scope/2, Sum3/2
  PI输出限幅1/1 -> Scope/1, ist*/1

== system trainn_traction_system_4motors_CRH3_ver1/motor module1/Subsystem1/转速调节器ASR ==
  "  " : Inport
  Integrator : Integrator
  I积分放大倍数 : Gain  Gain=0.08
  PI输出限幅2 : Saturate  UpperLimit=400  LowerLimit=-400
  P比例放大倍数 : Gain  Gain=12
  Scope : Scope  NumInputPorts=2
  Sum1 : Sum  Inputs=|++
  Te* : Outport  VectorParamsAs1DForOutWhenUnconnected=off
  wires:
  I积分放大倍数/1 -> Integrator/1
  "  "/1 -> I积分放大倍数/1, P比例放大倍数/1
  P比例放大倍数/1 -> Sum1/1
  Integrator/1 -> Scope/2, Sum1/2
  Sum1/1 -> PI输出限幅2/1
  PI输出限幅2/1 -> Scope/1, Te*/1

== system trainn_traction_system_4motors_CRH3_ver1/motor module2/Subsystem2/ACMR ==
  "  " : Inport
  Integrator : Integrator
  I积分放大倍数 : Gain  Gain=50
  PI输出限幅 : Saturate  UpperLimit=Vdc_ref/sqrt(6)  LowerLimit=-Vdc_ref/sqrt(6)
  P比例放大倍数 : Gain
  Scope : Scope  NumInputPorts=2
  Sum1 : Sum  Inputs=|++
  带限幅的连续积分1 : Integrator  LimitOutput=on  UpperSaturationLimit=390  LowerSaturationLimit=-390
  " " : Outport  VectorParamsAs1DForOutWhenUnconnected=off
  wires:
  Sum1/1 -> PI输出限幅/1
  PI输出限幅/1 -> " "/1, Scope/1
  P比例放大倍数/1 -> Sum1/1
  I积分放大倍数/1 -> Integrator/1
  "  "/1 -> I积分放大倍数/1, P比例放大倍数/1
  Integrator/1 -> Scope/2, Sum1/2

== system trainn_traction_system_4motors_CRH3_ver1/motor module2/Subsystem2/ACTR ==
  "  " : Inport
  Integrator : Integrator
  I积分放大倍数 : Gain  Gain=3.5
  PI输出限幅 : Saturate  UpperLimit=Vdc_ref/sqrt(6)  LowerLimit=-1*Vdc_ref/sqrt(6)
  PI输出限幅1 : Saturate  UpperLimit=Vdc_ref  LowerLimit=-1*Vdc_ref
  P比例放大倍数 : Gain  Gain=1.5
  Scope : Scope  NumInputPorts=2
  Sum1 : Sum  Inputs=|++
  带限幅的连续积分1 : Integrator  LimitOutput=on  UpperSaturationLimit=400  LowerSaturationLimit=-400
  " " : Outport  VectorParamsAs1DForOutWhenUnconnected=off
  wires:
  Sum1/1 -> PI输出限幅/1
  PI输出限幅/1 -> " "/1, Scope/1
  P比例放大倍数/1 -> Sum1/1
  I积分放大倍数/1 -> Integrator/1
  "  "/1 -> I积分放大倍数/1, P比例放大倍数/1
  Integrator/1 -> Scope/2, Sum1/2

== system trainn_traction_system_4motors_CRH3_ver1/motor module2/Subsystem2/SVPWM ==
  Udc : Inport
  Ualpha : Inport  Port=2
  Ubeta : Inport  Port=3
  " Gen Gate" : MATLAB Function  TreatAsAtomicUnit=on
  Clock : Clock
  Constant2 : Constant  Value=Ts
  Constant3 : Constant  Value=Ts
  Data Type Conversion : DataTypeConversion  OutDataTypeStr=boolean
  Delay{,1..4} (5 alike) : Delay  DelayLength=1  InitialCondition=0
  MATLAB Function1 : MATLAB Function  TreatAsAtomicUnit=on
  MATLAB Function3 : MATLAB Function  TreatAsAtomicUnit=on
  Pulse Generator : DiscretePulseGenerator  PulseType=Time based  Period=Ts
  Scope1 : Scope  NumInputPorts=3
  Scope3 : Scope
  find section1 : Subsystem
  g : Outport
  wires:
  Ualpha/1 -> find section1/1(Ualpha), MATLAB Function3/2(Ualpha)
  Pulse Generator/1 -> Data Type Conversion/1
  MATLAB Function1/2(newT0) -> " Gen Gate"/4(T0), Delay/1
  Delay1/1 -> MATLAB Function1/1(old_t0)
  MATLAB Function3/3(T2) -> Scope1/3, MATLAB Function1/6(T2)
  Ubeta/1 -> find section1/2(Ubeta), MATLAB Function3/3(Ubeta)
  find section1/1(section) -> MATLAB Function1/7(sec), MATLAB Function3/5(sec)
  Constant2/1 -> MATLAB Function3/4(Ts)
  MATLAB Function3/2(T1) -> Scope1/2, MATLAB Function1/5(T1)
  MATLAB Function1/1(new_t0) -> Scope3/1, Delay1/1, " Gen Gate"/2(t0)
  Clock/1 -> " Gen Gate"/1(t), MATLAB Function1/2(t)
  MATLAB Function3/1(T0) -> MATLAB Function1/4(T0), Scope1/1
  Constant3/1 -> " Gen Gate"/3(Ts)
  Udc/1 -> MATLAB Function3/1(Udc)
  " Gen Gate"/1(g) -> g/1
  Data Type Conversion/1 -> MATLAB Function1/3(trigger)
  MATLAB Function1/5(newSec) -> Delay2/1, " Gen Gate"/7(sec)
  Delay2/1 -> MATLAB Function1/11(oldSec)
  MATLAB Function1/4(newT2) -> Delay3/1, " Gen Gate"/6(T2)
  Delay3/1 -> MATLAB Function1/10(oldT2)
  MATLAB Function1/3(newT1) -> Delay4/1, " Gen Gate"/5(T1)
  Delay4/1 -> MATLAB Function1/9(oldT1)
  Delay/1 -> MATLAB Function1/8(oldT0)

== system trainn_traction_system_4motors_CRH3_ver1/motor module2/Subsystem2/SVPWM1 ==
  Udc : Inport
  Ualpha : Inport  Port=2
  Ubeta : Inport  Port=3
  Constant2 : Constant  Value=Tpwm
  Constant4 : Constant  Value=Tpwm
  MATLAB Function10 : MATLAB Function  TreatAsAtomicUnit=on
  MATLAB Function3 : MATLAB Function  TreatAsAtomicUnit=on
  Mux : Mux  Inputs=6
  Repeating Sequence1 : simulink/Sources/Repeating Sequence  rep_seq_t=[0 Tpwm]  rep_seq_y=[0 Tpwm]
  Scope1 : Scope  NumInputPorts=3
  find section1 : Subsystem
  g : Outport
  wires:
  Ualpha/1 -> find section1/1(Ualpha), MATLAB Function3/2(Ualpha)
  Ubeta/1 -> find section1/2(Ubeta), MATLAB Function3/3(Ubeta)
  Constant2/1 -> MATLAB Function3/4(Ts)
  MATLAB Function3/1(T0) -> Scope1/1
  Udc/1 -> MATLAB Function3/1(Udc)
  MATLAB Function3/2(T1) -> Scope1/2, MATLAB Function10/1(Ta)
  find section1/1(section) -> MATLAB Function10/4(section), MATLAB Function3/5(sec)
  Constant4/1 -> MATLAB Function10/3(Tpwm)
  Repeating Sequence1/1 -> MATLAB Function10/5(t)
  MATLAB Function3/3(T2) -> Scope1/3, MATLAB Function10/2(Tb)
  MATLAB Function10/6(gCN) -> Mux/6
  MATLAB Function10/5(gC) -> Mux/5
  MATLAB Function10/4(gBN) -> Mux/4
  MATLAB Function10/3(gB) -> Mux/3
  MATLAB Function10/2(gAN) -> Mux/2
  MATLAB Function10/1(gA) -> Mux/1
  Mux/1 -> g/1

== system trainn_traction_system_4motors_CRH3_ver1/motor module2/Subsystem2/Subsystem ==
  note: Tr = Lr / Rr
  note: phy_r
  note: ws
  note: w1
  id(im) : Inport
  iq(it) : Inport  Port=2
  w : Inport  Port=3
  Divide{,2..4} (4 alike) : Product  Inputs=/*
  Divide1 : Product  Inputs=*/
  Gain1 : Gain  Gain=Lm
  Gain2 : Gain  Gain=Lm
  Integrator1 : Integrator  InitialCondition=1e-5
  Integrator2 : Integrator
  Lr : Constant  Value=Llr + 1.5*Lm
  Rr : Constant  Value=Rr
  Scope3 : Scope  NumInputPorts=2
  Sum : Sum  Inputs=-+|
  Sum1 : Sum  Inputs=|++
  phi : Outport
  theta : Outport  Port=2
  wires:
  Divide/1 -> Sum1/1
  Divide3/1 -> Divide/2
  Sum/1 -> Integrator1/1
  iq(it)/1 -> Gain2/1, Scope3/2
  Sum1/1 -> Integrator2/1
  id(im)/1 -> Gain1/1, Scope3/1
  w/1 -> Sum1/2
  Integrator2/1 -> theta/1
  Lr/1 -> Divide1/1
  Rr/1 -> Divide1/2
  Divide2/1 -> Sum/2
  Gain1/1 -> Divide2/2
  Integrator1/1 -> Divide4/2, Divide/1, phi/1
  Divide4/1 -> Sum/1
  Divide1/1 -> Divide3/1, Divide2/1, Divide4/1
  Gain2/1 -> Divide3/2

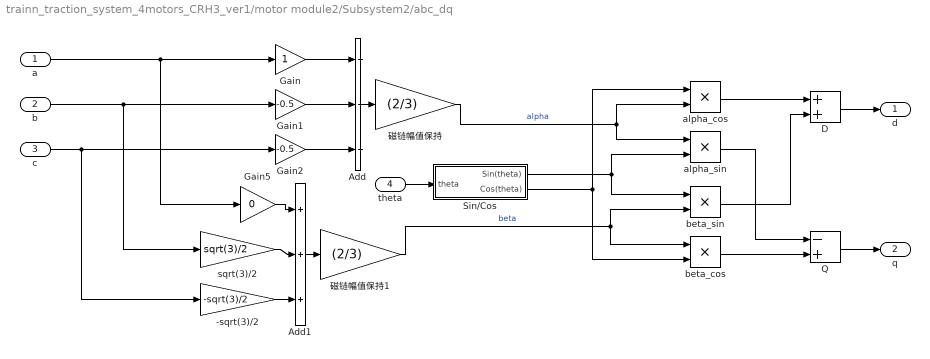
== system trainn_traction_system_4motors_CRH3_ver1/motor module2/Subsystem2/abc_dq ==
  a : Inport
  b : Inport  Port=2
  c : Inport  Port=3
  theta : Inport  Port=4
  -sqrt(3)/2 : Gain  Gain=-sqrt(3)/2
  Add : Sum  Inputs=3
  Add1 : Sum  Inputs=3
  D : Sum
  Gain : Gain
  Gain1 : Gain  Gain=-0.5
  Gain2 : Gain  Gain=-0.5
  Gain5 : Gain  Gain=0
  Q : Sum  Inputs=-+
  Sin/Cos : Subsystem
  alpha_cos : Product
  alpha_sin : Product
  beta_cos : Product
  beta_sin : Product
  sqrt(3)/2 : Gain  Gain=sqrt(3)/2
  磁链幅值保持 : Gain  Gain=(2/3)
  磁链幅值保持1 : Gain  Gain=(2/3)
  d : Outport  VectorParamsAs1DForOutWhenUnconnected=off
  q : Outport  Port=2  VectorParamsAs1DForOutWhenUnconnected=off
  wires:
  磁链幅值保持1/1 -> beta_cos/1, beta_sin/2  "beta"
  D/1 -> d/1
  Sin/Cos/2(Cos(theta)) -> beta_cos/2, alpha_cos/1
  alpha_sin/1 -> Q/1
  Q/1 -> q/1
  beta_sin/1 -> D/2
  beta_cos/1 -> Q/2
  Sin/Cos/1(Sin(theta)) -> beta_sin/1, alpha_sin/2
  磁链幅值保持/1 -> alpha_cos/2, alpha_sin/1  "alpha"
  Add1/1 -> 磁链幅值保持1/1
  c/1 -> Gain2/1, -sqrt(3)/2/1
  a/1 -> Gain5/1, Gain/1
  Gain2/1 -> Add/3
  sqrt(3)/2/1 -> Add1/2
  theta/1 -> Sin/Cos/1(theta)
  b/1 -> sqrt(3)/2/1, Gain1/1
  -sqrt(3)/2/1 -> Add1/3
  Gain1/1 -> Add/2
  Gain5/1 -> Add1/1
  alpha_cos/1 -> D/1
  Add/1 -> 磁链幅值保持/1
  Gain/1 -> Add/1

== system trainn_traction_system_4motors_CRH3_ver1/motor module2/Subsystem2/dq-alpha\beta1 ==
  Q : Inport
  D : Inport  Port=2
  theta : Inport  Port=3
  Product{,1..3} (4 alike) : Product
  Sum1 : Sum  Inputs=++|
  Sum3 : Sum  Inputs=|+-
  Trigonometric Function : Trigonometry
  Trigonometric Function1 : Trigonometry  Operator=cos
  alpha : Outport
  beta : Outport  Port=2
  wires:
  Sum1/1 -> beta/1
  Product3/1 -> Sum1/2
  Product2/1 -> Sum1/1
  Sum3/1 -> alpha/1
  Product1/1 -> Sum3/2
  Product/1 -> Sum3/1
  Trigonometric Function/1 -> Product1/1, Product2/1
  Trigonometric Function1/1 -> Product/2, Product3/1
  Q/1 -> Product1/2, Product3/2
  theta/1 -> Trigonometric Function/1, Trigonometric Function1/1
  D/1 -> Product2/2, Product/1

== system trainn_traction_system_4motors_CRH3_ver1/motor module2/Subsystem2/磁链调节器APhirR ==
  " " : Inport
  Integrator : Integrator
  I积分放大倍数 : Gain  Gain=3.6
  PI输出限幅1 : Saturate  UpperLimit=13  LowerLimit=-13
  P比例放大倍数 : Gain  Gain=1.8
  Scope : Scope  NumInputPorts=2
  Sum1 : Sum  Inputs=|++
  带限幅的连续积分1 : Integrator  LimitOutput=on  UpperSaturationLimit=15  LowerSaturationLimit=-15
  ism* : Outport  VectorParamsAs1DForOutWhenUnconnected=off
  wires:
  P比例放大倍数/1 -> Sum1/1
  " "/1 -> I积分放大倍数/1, P比例放大倍数/1
  Sum1/1 -> ism*/1, Scope/1
  I积分放大倍数/1 -> Integrator/1
  Integrator/1 -> Scope/2, Sum1/2
